simulink model "modelo"  (R2015a)
settings: Solver=ode3  StartTime=0.0  StopTime=10.0  RelTol=1e-3
undefined symbols (not defined in the file): a, b
libraries: simulink x1
settings Model: Creator=Denis  LastModifiedBy=Denis
settings OptimizationCC: OptimizeModelRefInitCode=on  LifeSpan=1  MaxStackSize=64
settings HardwareCC: ProdLargestAtomicInteger=Long  ProdLargestAtomicFloat=Double  ProdEndianess=LittleEndian  ProdHWDeviceType=ARM Compatible->ARM Cortex
settings RTWCC: SystemTargetFile=ert.tlc  TemplateMakefile=ert_default_tmf  Description=Embedded Coder  Toolchain=GNU Tools for ARM Embedded Processors  CreateSILPILBlock=PIL
settings CodeAppCC: IgnoreCustomStorageClasses=off
settings ERTTargetCC: GenerateSampleERTMain=off  ParMdlRefBuildCompliant=on  CompOptLevelCompliant=on  ConcurrentExecutionCompliant=on  ERTFirstTimeCompliant=on  SupportContinuousTime=off  SupportVariableSizeSignals=off  ModelStepFunctionPrototypeControlCompliant=on  CPPClassGenCompliant=on  InlinedParameterPlacement=Hierarchical

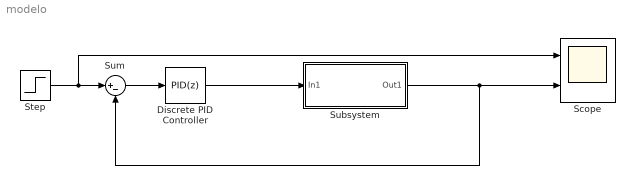
== system modelo ==
  Discrete PID Controller : simulink/Continuous/PID Controller  Controller=PID  TimeDomain=Discrete-time  SampleTime=0.01  IntegratorMethod=Forward Euler  FilterMethod=Forward Euler  Form=Parallel  UseFilter=off  ControllerParametersSource=internal  P=2.44125432515755  I=0.894522737934024  D=1.48874538196239  N=37.5163389731792  InitialConditionSource=internal  InitialConditionForIntegrator=0  InitialConditionForFilter=0  ExternalReset=none  LimitOutput=off  UpperSaturationLimit=inf  LowerSaturationLimit=-inf  LinearizeAsGain=off  AntiWindupMode=none  Kb=1  TrackingMode=off  Kt=1  PParamMin=[]  PParamMax=[]  IParamMin=[]  IParamMax=[]  DParamMin=[]  DParamMax=[]  NParamMin=[]  NParamMax=[]  KbParamMin=[]  KbParamMax=[]  KtParamMin=[]  KtParamMax=[]  POutMin=[]  POutMax=[]  IOutMin=[]  IOutMax=[]  DOutMin=[]  DOutMax=[]  NOutMin=[]  NOutMax=[]  KbOutMin=[]  KbOutMax=[]  KtOutMin=[]  KtOutMax=[]  IntegratorOutMin=[]  IntegratorOutMax=[]  FilterOutMin=[]  FilterOutMax=[]  SumOutMin=[]  SumOutMax=[]  SumI1OutMin=[]  SumI1OutMax=[]  SumI2OutMin=[]  SumI2OutMax=[]  SumI3OutMin=[]  SumI3OutMax=[]  SumDOutMin=[]  SumDOutMax=[]  SaturationOutMin=[]  SaturationOutMax=[]  IntegratorContinuousStateAttributes=''  IntegratorStateMustResolveToSignalObject=off  IntegratorRTWStateStorageClass=Auto  FilterContinuousStateAttributes=''  FilterStateMustResolveToSignalObject=off  FilterRTWStateStorageClass=Auto  DifferentiatorICPrevScaledInput=0  DifferentiatorOutMin=[]  DifferentiatorOutMax=[]
  Scope : Scope  NumInputPorts=2
      settings: YMin=-5~-5  YMax=5~5
  Step : Step  Time=0  SampleTime=0
  Subsystem : Subsystem
  Sum : Sum  Inputs=|+-
  wires:
  Sum/1 -> Discrete PID Controller/1
  Subsystem/1(Out1) -> Scope/2, Sum/2
  Step/1 -> Scope/1, Sum/1
  Discrete PID Controller/1 -> Subsystem/1(In1)

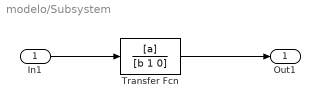
== system modelo/Subsystem ==
  In1 : Inport
  Transfer Fcn : TransferFcn  Numerator=[a]  Denominator=[b 1 0]
  Out1 : Outport
  wires:
  Transfer Fcn/1 -> Out1/1
  In1/1 -> Transfer Fcn/1
